simulink model "MicrochipTargetMotorControl"  (R2024b)
settings: Solver=FixedStepDiscrete  StartTime=0.0  StopTime=50  RelTol=1e-3  EnableMultiTasking=on
InitFcn:
  | MicrochipTargetMotorControlData;
  | mcbMotorSwapData;
values from neighbouring files (symbols this model uses):
  Ts = T_pwm    [mcbMotorSwapData.m]
  Ts_motor = T_pwm/2    [mcbMotorSwapData.m]
  Ts_serialIn = 50e-3    (= 0.05)    [MicrochipTargetMotorControlData.m]
  Ts_speed = 10*Ts    [mcbMotorSwapData.m]
undefined symbols (not defined in the file or in its folder): A4, B0, C10, C11, C6, C7, C8, inverter, MaxPer, P17, P20, P39, P40, P41, P43, P44, Pin, pmsm, Resol, s, target, Timer, us
libraries: MCHP_Blockset x19, simulink x13, autolibpmsminterior x1, mcbplantlib x1, mcbcontrolslib x1
(part 4 of 4)

== system MicrochipTargetMotorControl/Microcontroller/OutputHWDrivers/codegen ==
  PWMIn : Inport
  InverterEn : Inport  Port=2
  Ground : Ground
  NOT : Logic  Operator=NOT  IconShape=distinctive  AllPortsSameDT=off  OutDataTypeStr=boolean
  PWMDisable : Subsystem
  PWMEnable : Subsystem
  PWM_HS_FEP : MCHP_Blockset/PWM IO/PWM_HS_FEP  Priority=-2000  PWMx_MODSEL=Center Aligned  PWMx_CLKSEL=no scaling  PWM_ClockResolution_DIVSEL_TXT=auto  PWM_ClockResolution_FSCL_TXT="Resol: 0.275(us)  -  MaxPer: 0.018(s)"  PWM_ClockResolution_NoScaling_TXT="Resol: 0.005(us)  -  MaxPer: 0.000328(s)"  MaxPeriod_s=Ts  InitPeriode_s=Ts  InitDutyCycleP_s=0  InitDutyCycleS_s=10e-6  InitPhase_s=-1  evalin_ws=PWM1max=MCHP_Fun.Hex2num('40B86A0000000000');PWM2max=MCHP_Fun.Hex2num('40B86A0000000000');PWM3max=MCHP_Fun.Hex2num('40B86A0000000000');  SampleTime=-1  S_INPUT=[-1]  S_INPUT_Size=[3]  S_OUTPUT=[]  S_OUTPUT_Size=[]  S_ListCustomDatatype=S.S_ListCustomDatatype={};  MCHP_USER_INTERRUPTS=0  MCHP_PORT={PWMH1 }{PWMH1}32:4:D2;{PWMH2 }{PWMH2}32:4:D0;{PWMH3 }{PWMH3}32:4:C3;{PWML1}{PWML1}32:4:D3;{PWML2}{PWML2}32:4:D1;{PWML3}{PWML3}32:4:C4;  MCHP_MASTERLINK=MicrochipTargetMotorControl/Microcontroller/HWConfigurations/Microchip Master  MCHP_CRC=4877994  PWMx_PMOD=Complementary  PWM1_HL=PWMxH & PWMxL output enabled  PWM1_swap=off  PWM1H_pol=off  PWM1L_pol=off  PWM2_HL=PWMxH & PWMxL output enabled  PWM2_swap=off  PWM2H_pol=off  PWM2L_pol=off  PWM3_HL=PWMxH & PWMxL output enabled  PWM3_swap=off  PWM3H_pol=off  PWM3L_pol=off  PWM4_HL=not used  PWM4_swap=off  PWM4H_pol=off  PWM4L_pol=off  PWM5_HL=not used  PWM5_swap=off  PWM5H_pol=off  PWM5L_pol=off  PWM6_HL=not used  PWM6_swap=off  PWM6H_pol=off  PWM6L_pol=off  PWM7_HL=not used  PWM7_swap=off  PWM7H_pol=off  PWM7L_pol=off  PWM8_HL=not used  PWM8_swap=off  PWM8H_pol=off  PWM8L_pol=off  PWM9_HL=not used  PWM9_swap=off  PWM9H_pol=off  PWM9L_pol=off  PWM10_HL=not used  PWM10_swap=off  PWM10H_pol=off  PWM10L_pol=off  PWM11_HL=not used  PWM11_swap=off  PWM11H_pol=off  PWM11L_pol=off  PWM12_HL=not used  PWM12_swap=off  PWM12H_pol=off  PWM12L_pol=off  PWM1_ShowTrig=on  PWM1_Init_PGxTRIGABC_s=[0 -1 -1 ]  PWM1_ADTRxEN1=ADC Trigger 1  PWM1_ADTRxEN2=none  PWM1_ADTRxEN3=none  PWM2_ShowTrig=off  PWM2_Init_PGxTRIGABC_s=[-1 -1 -1]  PWM2_ADTRxEN1=none  PWM2_ADTRxEN2=none  PWM2_ADTRxEN3=none  PWM3_ShowTrig=off  PWM3_Init_PGxTRIGABC_s=[-1 -1 -1]  PWM3_ADTRxEN1=none  PWM3_ADTRxEN2=none  PWM3_ADTRxEN3=none  PWM4_ShowTrig=off  PWM4_Init_PGxTRIGABC_s=[-1 -1 -1]  PWM4_ADTRxEN1=none  PWM4_ADTRxEN2=none  PWM4_ADTRxEN3=none  PWM5_ShowTrig=off  PWM5_Init_PGxTRIGABC_s=[-1 -1 -1]  PWM5_ADTRxEN1=none  PWM5_ADTRxEN2=none  PWM5_ADTRxEN3=none  PWM6_ShowTrig=off  PWM6_Init_PGxTRIGABC_s=[-1 -1 -1]  PWM6_ADTRxEN1=none  PWM6_ADTRxEN2=none  PWM6_ADTRxEN3=none  PWM7_ShowTrig=off  PWM7_Init_PGxTRIGABC_s=[-1 -1 -1]  PWM7_ADTRxEN1=none  PWM7_ADTRxEN2=none  PWM7_ADTRxEN3=none  PWM8_ShowTrig=off  PWM8_Init_PGxTRIGABC_s=[-1 -1 -1]  PWM8_ADTRxEN1=none  PWM8_ADTRxEN2=none  PWM8_ADTRxEN3=none  BlockInput_VectorScalar=Vectors (grouped by function)  BlockInput_Period=Not a block input  BlockInput_DutyCycle=a Floating Point input within range [0 1]  BlockInput_PhaseShift=Not a block input  BlockInput_SEVTCMP=Not a block input  BlockInput_TRIGx=Not a block input  BlockInput_DeadTime=Not a block input  BlockOutput_FaultDisabled=off  BlockOutput_Fault=on  DTC=Positive dead time (ensure period of time with PWM_H and PWM_L disasserted)  FLTSRC1_DTCMP_TXT=<empty>  FLTSRC2_DTCMP_TXT=<empty>  FLTSRC3_DTCMP_TXT=<empty>  FLTSRC4_DTCMP_TXT=<empty>  FLTSRC5_DTCMP_TXT=<empty>  FLTSRC6_DTCMP_TXT=<empty>  FLTSRC7_DTCMP_TXT=<empty>  FLTSRC8_DTCMP_TXT=<empty>  FLTSRC9_DTCMP_TXT=<empty>  FLTSRC10_DTCMP_TXT=<empty>  FLTSRC11_DTCMP_TXT=<empty>  FLTSRC12_DTCMP_TXT=<empty>  DeadTime_s=2e-6  DeadTimeAlt_s=2e-6  DeadTimeComp_s=0  FLTMODx=Disabled  FLTSRCx_TXT=<empty>  FLTDATx=PWM H/L -> 11  CLMODx=Disabled  CLSRCx_TXT=<empty>  CLDATx=PWM H/L -> 00  FLTLEBENx=off  CLLEBENx=off  LeadEdgeBlkPer_s=5e-7  PHRx=off  PHFx=off  PLRx=off  PLFx=off
      settings: SourceProductName=MPLAB Device Blocks for Simulink
  PWMDutyCycles : Outport
  wires:
  PWMIn/1 -> PWM_HS_FEP/1
  Ground/1 -> PWMDutyCycles/1
  InverterEn/1 -> NOT/1, PWMEnable/Enable
  NOT/1 -> PWMDisable/Enable

== system MicrochipTargetMotorControl/Microcontroller/OutputHWDrivers/sim ==
  PWMIn : Inport
  InverterEn : Inport  Port=2
  Terminator : Terminator
  PWMDutyCycles : Outport
  wires:
  InverterEn/1 -> Terminator/1
  PWMIn/1 -> PWMDutyCycles/1

== system MicrochipTargetMotorControl/Microcontroller/SerialInDrivers/Triggered Subsystem ==
  In1 : Inport
  Trigger : TriggerPort  VariantControl=(inherit)
  SCI_Data : Outport
  wires:
  In1/1 -> SCI_Data/1

== system MicrochipTargetMotorControl/Microcontroller/SerialOutDrivers/codegen ==
  SerialData : Inport
  Serial_Tx : Subsystem
  wires:
  SerialData/1 -> Serial_Tx/1(Data_Log)

== system MicrochipTargetMotorControl/Microcontroller/SerialOutDrivers/sim ==
  SerialData : Inport
  Terminator : Terminator
  wires:
  SerialData/1 -> Terminator/1

== system MicrochipTargetMotorControl/Inverter and Motor/sim/Motor/Inverter ==
  Duty_abc : Inport
  Average-Value Inverter : mcbplantlib/Average-Value Inverter
  Constant2 : Constant  Value=inverter.V_dc  OutDataTypeStr=single  SampleTime=-1
  Data Type Conversion1 : DataTypeConversion  OutDataTypeStr=single  RndMeth=Simplest  SaturateOnIntegerOverflow=off
  Rate Transition3 : RateTransition  Deterministic=off  OutPortSampleTime=Ts_inverter
  Vabc : Outport  VectorParamsAs1DForOutWhenUnconnected=off
  wires:
  Constant2/1 -> Average-Value Inverter/2
  Data Type Conversion1/1 -> Rate Transition3/1
  Duty_abc/1 -> Data Type Conversion1/1
  Rate Transition3/1 -> Average-Value Inverter/1
  Average-Value Inverter/1 -> Vabc/1

== system MicrochipTargetMotorControl/Inverter and Motor/sim/Motor/Load_Profile (Torque) ==
  IIR Filter : mcbcontrolslib/IIR Filter  VariantControl=Low Pass Filter  VariantSelect=Low-pass  FilterConstantInputType=Specify via dialog  Filter_constant=0.0001  advancedSettings=off  Ts=50e-6  cutOff_freq=0.31834
  T_load : Step  Time=8  After=0.05 * pmsm.T_rated  SampleTime=Ts_motor
  Load_Trq : Outport  VectorParamsAs1DForOutWhenUnconnected=off
  wires:
  T_load/1 -> IIR Filter/1
  IIR Filter/1 -> Load_Trq/1  "LoadTorque"

== system MicrochipTargetMotorControl/Inverter and Motor/sim/Sensor_Measurements/Get_PU  ==
  rad : Inport
  Constant2 : Constant  Value=2*pi  OutDataTypeStr=single  SampleTime=-1
  Get_PU : Gain  Gain=1/(2*pi)  OutDataTypeStr=dataType  RndMeth=Simplest
  Mod : Math  Operator=mod
  PU : Outport  VectorParamsAs1DForOutWhenUnconnected=off
  wires:
  Mod/1 -> Get_PU/1
  Constant2/1 -> Mod/2
  rad/1 -> Mod/1
  Get_PU/1 -> PU/1

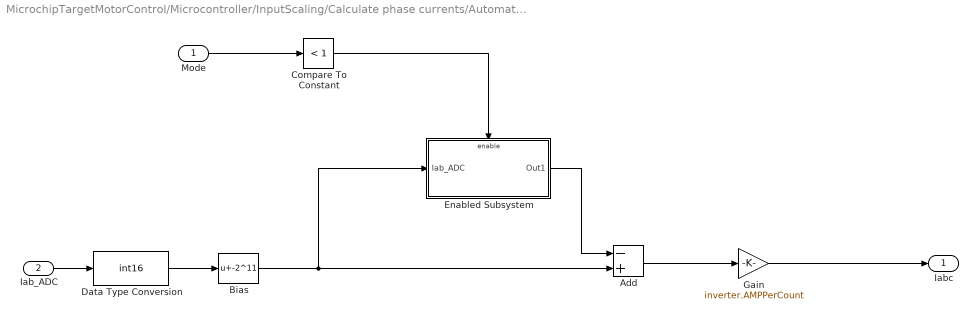
== system MicrochipTargetMotorControl/Microcontroller/InputScaling/Calculate phase currents/Automatic offset calibration ==
  Mode : Inport
  Iab_ADC : Inport  Port=2
  Add : Sum  Inputs=-+
  Bias : Bias  Bias=-2^11  SaturateOnIntegerOverflow=off
  Compare To Constant : simulink/Logic and Bit Operations/Compare To Constant  relop=<  const=1  OutDataTypeStr=boolean
  Data Type Conversion : DataTypeConversion  OutDataTypeStr=int16  SaturateOnIntegerOverflow=off  RndMeth=Floor
  Enabled Subsystem : Subsystem  TreatAsAtomicUnit=on
  Gain : Gain  Gain=inverter.AMPPerCount  OutDataTypeStr=dataType  RndMeth=Simplest
  Iabc : Outport
  wires:
  Mode/1 -> Compare To Constant/1
  Compare To Constant/1 -> Enabled Subsystem/Enable
  Iab_ADC/1 -> Data Type Conversion/1
  Add/1 -> Gain/1
  Enabled Subsystem/1(Out1) -> Add/1
  Bias/1 -> Add/2, Enabled Subsystem/1(Iab_ADC)
  Gain/1 -> Iabc/1
  Data Type Conversion/1 -> Bias/1

== system MicrochipTargetMotorControl/Microcontroller/InputScaling/Calculate phase currents/Offser via parameter ==
  Mode : Inport
  Iab_ADC : Inport  Port=2
  Add : Sum  Inputs=-+
  Constant : Constant  Value=[inverter.CtSensAOffset inverter.CtSensBOffset]  OutDataTypeStr=int16
  Gain : Gain  Gain=inverter.AMPPerCount  OutDataTypeStr=dataType  RndMeth=Simplest
  Terminator : Terminator
  Iabc : Outport
  wires:
  Mode/1 -> Terminator/1
  Iab_ADC/1 -> Add/2
  Constant/1 -> Add/1
  Add/1 -> Gain/1
  Gain/1 -> Iabc/1

== system MicrochipTargetMotorControl/Microcontroller/OutputHWDrivers/codegen/PWMDisable ==
  Enable : EnablePort
  C Function Call : MCHP_Blockset/User Functions/C Function Call  ParseFilesChkbx=off  ListFunctions1=Custom Function  Function1=void DisablePWMOutputs(void);  AddHeaderDeclaration=off  Function1Type=when block is updated (default)  FctReturnBlockOut=off  DataCollected=0  ORDERING=None  SampleTime=-1  S_INPUT=0  S_INPUT_Size=0  S_OUTPUT=0  S_OUTPUT_Size=0  S_ListCustomDatatype=0  MCHP_CRC=1011822  MCHP_MASTERLINK=MicrochipTargetMotorControl/Microcontroller/HWConfigurations/Microchip Master  PinDigitalInput=[]  PinDigitalOutput=[]  PinAnalogInput=[]
      settings: SourceProductName=MPLAB Device Blocks for Simulink

== system MicrochipTargetMotorControl/Microcontroller/OutputHWDrivers/codegen/PWMEnable ==
  Enable : EnablePort
  C Function Call1 : MCHP_Blockset/User Functions/C Function Call  ParseFilesChkbx=off  ListFunctions1=Custom Function  Function1=void EnablePWMOutputs(void);  AddHeaderDeclaration=off  Function1Type=when block is updated (default)  FctReturnBlockOut=off  DataCollected=0  ORDERING=None  SampleTime=-1  S_INPUT=0  S_INPUT_Size=0  S_OUTPUT=0  S_OUTPUT_Size=0  S_ListCustomDatatype=0  MCHP_CRC=1004094  MCHP_MASTERLINK=MicrochipTargetMotorControl/Microcontroller/HWConfigurations/Microchip Master  PinDigitalInput=[]  PinDigitalOutput=[]  PinAnalogInput=[]
      settings: SourceProductName=MPLAB Device Blocks for Simulink

== system MicrochipTargetMotorControl/Microcontroller/SerialOutDrivers/codegen/Serial_Tx ==
  note: Fast Serial Data Monitoring (32-bit)
  Data_Log : Inport
  Constant : Constant  Value=target.frameSize -1  OutDataTypeStr=uint16
  Counter Limited : simulink/Sources/Counter Limited  uplimit=target.frameSize-1  tsamp=-1
  Data : Subsystem  TreatAsAtomicUnit=on
  Data Type Conversion : DataTypeConversion  OutDataTypeStr=uint16  RndMeth=Simplest  SaturateOnIntegerOverflow=off
  End : Subsystem  TreatAsAtomicUnit=on
  If : If  NumInputs=2  IfExpression=u1 == 0  ElseIfExpressions=u1 == u2
  Start : Subsystem  TreatAsAtomicUnit=on
  wires:
  If/3 -> Data/Action
  Counter Limited/1 -> Data Type Conversion/1
  If/2 -> End/Action
  If/1 -> Start/Action
  Data_Log/1 -> End/1(Data), Start/1(Data), Data/1(Data)
  Constant/1 -> If/2
  Data Type Conversion/1 -> If/1

== system MicrochipTargetMotorControl/Microcontroller/InputScaling/Calculate phase currents/Automatic offset calibration/Enabled Subsystem ==
  Iab_ADC : Inport
  Enable : EnablePort
  Out1 : Outport
  wires:
  Iab_ADC/1 -> Out1/1

== system MicrochipTargetMotorControl/Microcontroller/SerialOutDrivers/codegen/Serial_Tx/Data ==
  Data : Inport
  Action Port : ActionPort  ActionPortLabel=else
  UART Tx : MCHP_Blockset/BUS UART/UART Tx  UART_REF=1  ORDERING=None  AllOrNothing=off  SampleTime=-1  MCHP_MASTERLINK=MicrochipTargetMotorControl/Microcontroller/HWConfigurations/Microchip Master  NSend_Input=off  UART_String=off  NSend_Output=off
      settings: SourceProductName=MPLAB Device Blocks for Simulink
  wires:
  Data/1 -> UART Tx/1

== system MicrochipTargetMotorControl/Microcontroller/SerialOutDrivers/codegen/Serial_Tx/End ==
  Data : Inport
  Action Port : ActionPort  ActionPortLabel=elseif(u1 == u2)
  Mux : Mux  Inputs=2
  Start : Constant  Value=hex2dec('45')  OutDataTypeStr=uint8
  UART Tx : MCHP_Blockset/BUS UART/UART Tx  UART_REF=1  ORDERING=None  AllOrNothing=off  SampleTime=-1  MCHP_MASTERLINK=MicrochipTargetMotorControl/Microcontroller/HWConfigurations/Microchip Master  NSend_Input=off  UART_String=off  NSend_Output=off
      settings: SourceProductName=MPLAB Device Blocks for Simulink
  wires:
  Mux/1 -> UART Tx/1
  Data/1 -> Mux/1
  Start/1 -> Mux/2

== system MicrochipTargetMotorControl/Microcontroller/SerialOutDrivers/codegen/Serial_Tx/Start ==
  Data : Inport
  Action Port : ActionPort  ActionPortLabel=if(u1 == 0)
  End : Constant  Value=hex2dec('53')  OutDataTypeStr=uint8
  Mux : Mux  Inputs=2
  UART Tx : MCHP_Blockset/BUS UART/UART Tx  UART_REF=1  ORDERING=None  AllOrNothing=off  SampleTime=-1  MCHP_MASTERLINK=MicrochipTargetMotorControl/Microcontroller/HWConfigurations/Microchip Master  NSend_Input=off  UART_String=off  NSend_Output=off
      settings: SourceProductName=MPLAB Device Blocks for Simulink
  wires:
  Mux/1 -> UART Tx/1
  Data/1 -> Mux/2
  End/1 -> Mux/1
